simulink model "AnalogFilter"  (R2019b)
settings: Solver=VariableStepAuto  StartTime=0.0  StopTime=10.0  RelTol=1e-3
libraries: dsparch4 x4
settings Model: Creator=vezr2203  LastModifiedBy=lavc2115
settings SFSimCC: CustomCodeUndefinedFunction=UseInterfaceOnly

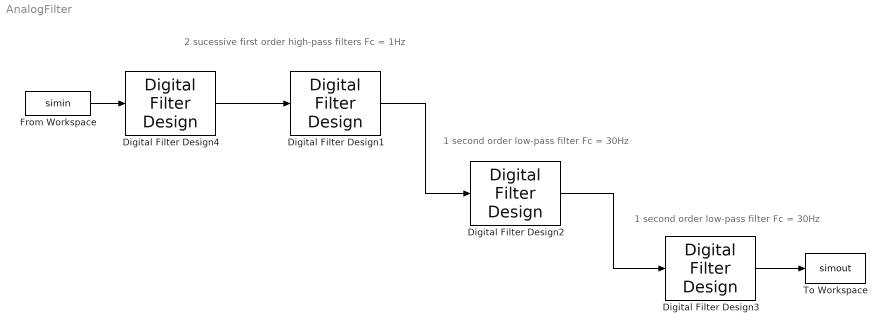
== system AnalogFilter ==
  note: 2 sucessive first order high-pass filters Fc = 1Hz
  note: 1 second order low-pass filter Fc = 30Hz
  note: 1 second order low-pass filter Fc = 30Hz
  Digital Filter Design{1..4} (4 alike) : dsparch4/Digital Filter Design  mwdsp_browser_bugfix_var=off
  From Workspace : FromWorkspace  VariableName=simin  SampleTime=1/250
  To Workspace : ToWorkspace  VariableName=simout  SaveFormat=Timeseries  SampleTime=1/250
  wires:
  Digital Filter Design4/1 -> Digital Filter Design1/1
  Digital Filter Design1/1 -> Digital Filter Design2/1
  Digital Filter Design2/1 -> Digital Filter Design3/1
  From Workspace/1 -> Digital Filter Design4/1
  Digital Filter Design3/1 -> To Workspace/1
